simulink model "main"  (R2015a)
settings: Solver=ode45  StartTime=0.0  StopTime=20  RelTol=1e-3
values from neighbouring files (symbols this model uses):
  s = tf('s')    [test.m]
libraries: slctrlblks x1
settings Model: Creator=christian  LastModifiedBy=christian

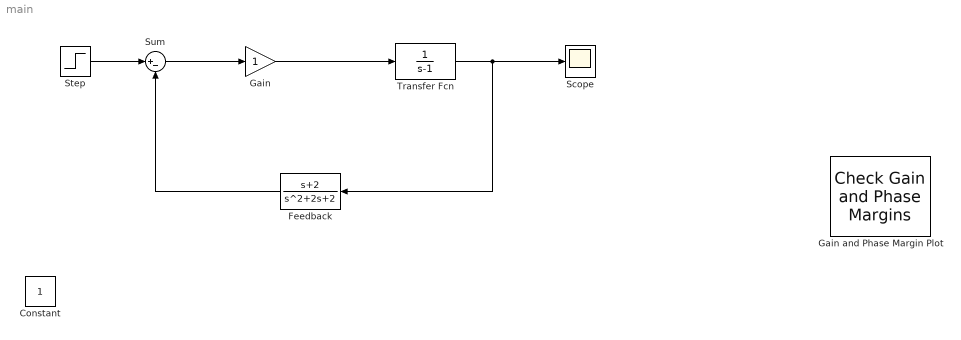
== system main ==
  Constant : Constant
  Feedback : TransferFcn  Numerator=[1 2]  Denominator=[1 2 2]
  Gain : Gain
  Gain and Phase Margin Plot : slctrlblks/Model Verification/Check Gain and Phase Margins  InstantiateOnLoad=on  SaveOperatingPoints=off  LinearizationIOs={'/Transfer Fcn', 1, 'out', 'off', '';'/Step', 1, 'in', 'off', ''}  LinearizeAt=SnapshotTimes  SnapshotTimes=[0]  TriggerType=rising  SampleTime=auto  RateConversionMethod=zoh  PreWarpFreq=10  UseExactDelayModel=off  UseFullBlockNameLabels=off  UseBusSignalLabels=off  enabled=on  stopWhenAssertionFail=off  export=off  ViewDlgPos=[100 200 510 390]  LaunchViewOnOpen=off  OpenViewOnLoad=off  FrequencyUnits=rad/s  MagnitudeUnits=dB  PhaseUnits=deg  TimeUnits=seconds  EnableMargins=off  GainMargin=[]  PhaseMargin=[]  PlotType=bode  FeedbackSign=-1
      settings: SaveToWorkspace=off  SaveName=sys
  Scope : Scope
  Step : Step  SampleTime=0
  Sum : Sum  Inputs=|+-
  Transfer Fcn : TransferFcn  Denominator=[1 -1]
  wires:
  Feedback/1 -> Sum/2
  Gain/1 -> Transfer Fcn/1
  Sum/1 -> Gain/1
  Transfer Fcn/1 -> Scope/1, Feedback/1
  Step/1 -> Sum/1
